simulink model "RCcircuit"  (R2018a)
settings: Solver=VariableStepAuto  StartTime=0.0  StopTime=10  RelTol=1e-3
libraries: pePwmGenerator x1, vrlib x1
settings Model: Creator=Ruben  LastModifiedBy=Ruben

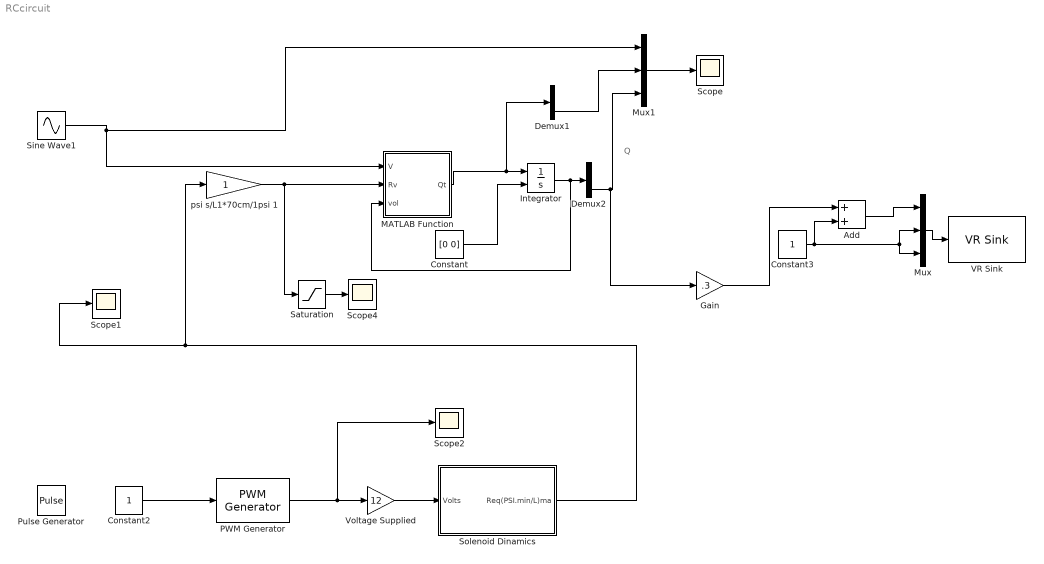
== system RCcircuit ==
  note: Q
  Add : Sum
  Constant : Constant  Value="[0    0]"
  Constant2 : Constant
  Constant3 : Constant
  Demux1 : Demux  Outputs=2
  Demux2 : Demux  Outputs=2
  Gain : Gain  Gain=.3
  Integrator : Integrator  InitialConditionSource=external
  MATLAB Function : MATLAB Function  TreatAsAtomicUnit=on
  Mux : Mux  Inputs=3
  Mux1 : Mux  Inputs=3
  PWM Generator : pePwmGenerator/PWM Generator  CarrCount=Up  Tper=0.1  Ts=5e-5
  Pulse Generator : DiscretePulseGenerator  PulseType=Time based  Period=3  PulseWidth=20
  Saturation : Saturate  UpperLimit=10
  Scope{,1..2,4} (4 alike) : Scope
  Sine Wave1 : Sin  Amplitude=2.5  Frequency=1.57  SampleTime=0
  Solenoid Dinamics : Subsystem  TreatAsAtomicUnit=on
  VR Sink : vrlib/VR Sink  InstantiateOnLoad=on  SampleTime=0.1  ViewEnable=on  RemoteChange=off  RemoteView=off  FieldsWritten=lungs.scale.3.1.1.double  WorldFileName=Lungs2.wrl  AutoView=off  VideoDimensions=[]  AllowVariableSize=off  FigureProperties="{'Position', 'Name', 'Viewpoint', 'CameraBound', 'CameraDirection', 'CameraPosition', 'CameraUpVector', 'ZoomFactor', 'Antialiasing', 'Headlight', 'Lighting', 'NavPanel', 'Sound', 'StatusBar', 'Stereo3D', 'Stereo3DCameraOffset', 'Stereo3DHIT', 'ToolBar', 'Textures', 'Transparency', 'Triad', 'Wireframe', 'NavZones', 'NavMode', 'NavSpeed', 'CaptureFileFormat', 'CaptureFileName', 'Record2DCompressMethod', 'Record2DCompressQuality', 'Record2D', 'Record2DFileName', 'Record2DFPS'; [1.4910000000000000e+03   1.5700000000000000e+02   5.7600000000000000e+02   3.5000000000000000e+02], '', 'DefaultViewpoint', 'on', [0.0000000000000000e+00   0.0000000000000000e+00  -1.0000000000000000e+00], [0.0000000000000000e+00   0.0000000000000000e+00   0.0000000000000000e+00], [0.0000000000000000e+00   1.0000000000000000e+00   0.0000000000000000e+00], [1.0000000000000000e+00], 'on', 'on', 'on', 'halfbar', 'on', 'on', 'off', [1.0000000149011612e-01], [0.0000000000000000e+00], 'on', 'on', 'on', 'none', 'off', 'off', 'fly', 'normal', 'tif', '%f_anim_%n.tif', 'auto', [7.5000000000000000e+01], 'off', '%f_anim_%n.avi', 'auto'}"
      settings: SourceProductBaseCode=VR
  Voltage Supplied : Gain  Gain=12
  psi s/L1*70cm/1psi 1 : Gain
  wires:
  MATLAB Function/1(Qt) -> Demux1/1, Integrator/1
  Integrator/1 -> Demux2/1, MATLAB Function/3(vol)
  Constant/1 -> Integrator/2
  Voltage Supplied/1 -> Solenoid Dinamics/1("Volts ")
  PWM Generator/1 -> Scope2/1, Voltage Supplied/1
  ? -> ?
  Solenoid Dinamics/1(Req(PSI.min/L)ma) -> Scope1/1, psi s/L1*70cm/1psi 1/1
  psi s/L1*70cm/1psi 1/1 -> Saturation/1, MATLAB Function/2(Rv)
  Saturation/1 -> Scope4/1
  Constant2/1 -> PWM Generator/1
  Sine Wave1/1 -> Mux1/1, MATLAB Function/1(V)
  Mux/1 -> VR Sink/1
  Constant3/1 -> Mux/3, Mux/2, Add/2
  Add/1 -> Mux/1
  Gain/1 -> Add/1
  Demux2/2 -> Gain/1, Mux1/3
  ? -> ?
  Mux1/1 -> Scope/1
  Demux1/2 -> Mux1/2

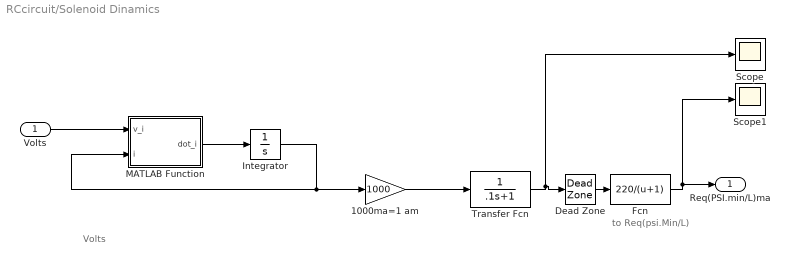
== system RCcircuit/Solenoid Dinamics ==
  note: to Req(psi.Min/L)
  note: Volts
  "Volts " : Inport
  1000ma=1 am : Gain  Gain=1000
  Dead Zone : DeadZone  LowerValue=0  UpperValue=200  SaturateOnIntegerOverflow=on
  Fcn : Fcn  Expr=220/(u+1)
  Integrator : Integrator
  MATLAB Function : MATLAB Function  TreatAsAtomicUnit=on
  Scope : Scope
  Scope1 : Scope
  Transfer Fcn : TransferFcn  Denominator=[.1 1]
  Req(PSI.min/L)ma : Outport
  wires:
  Integrator/1 -> 1000ma=1 am/1, MATLAB Function/2(i)
  MATLAB Function/1(dot_i) -> Integrator/1
  "Volts "/1 -> MATLAB Function/1(v_i)
  1000ma=1 am/1 -> Transfer Fcn/1
  Fcn/1 -> Scope1/1, Req(PSI.min/L)ma/1
  Dead Zone/1 -> Fcn/1
  Transfer Fcn/1 -> Dead Zone/1, Scope/1

== matlab function RCcircuit/Solenoid Dinamics/MATLAB Function ==
  data: v_i input; dot_i output; i input
function dot_i = fcn(v_i,i)
R=15; % R igual a 2 ohm
%L=.063 ;% L aprox 63mh
L=.063;
dot_i = (1/L)*(v_i-R*i);

== matlab function RCcircuit/MATLAB Function ==
  data: V input; Rv input; Qt output; vol input
function Qt  = fcn(V,Rv,vol)
intI2=vol(1);
intI3=vol(2);
Rc=1;Rp=1; %R1=RC,R2=Rp
Cs=.005;Cl=0.2; Cw=0.2;%C1=Cs; C2=Cl*CW
%Q=I3,Qa=I2



%C2=Cl+Cw
Q=(1/(Rc+Rv))*(V-(1/Cs)*(-intI2+intI3));
Qa=(1/Rp)*(V-Q*(Rc+Rv)-(1/(Cl+Cw))*intI2);

Qt = [ Qa  Q];
